simulink model "ej0311_PID"  (R2023b)
settings: Solver=VariableStepAuto  StartTime=0.0  StopTime=30  RelTol=1e-3
libraries: simulink x3
settings Model: Creator=cjuar  LastModifiedBy=cjuar

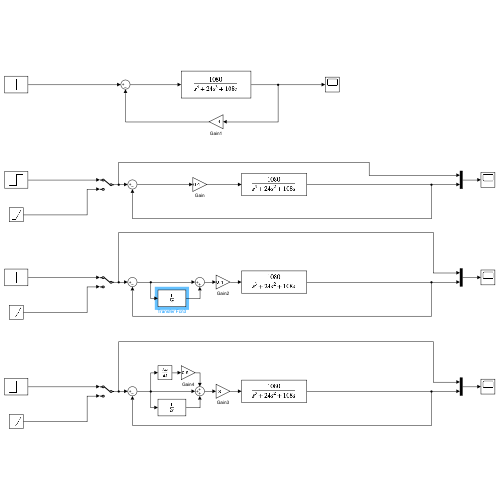
[thumbnail: Simulink's stored preview of the top-level diagram]
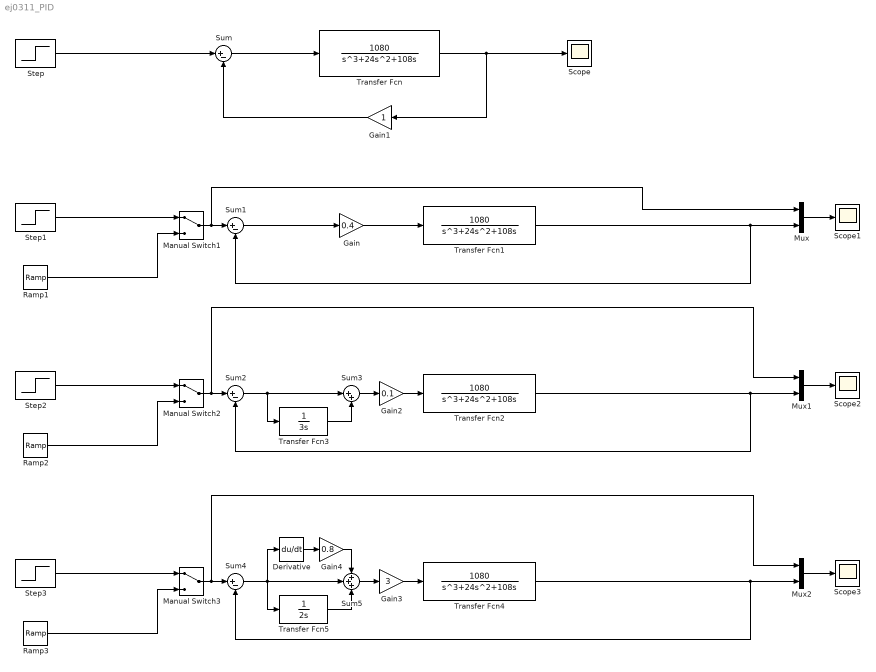
== system ej0311_PID ==
  Derivative : Derivative
  Gain : Gain  Gain=0.4
  Gain1 : Gain
  Gain2 : Gain  Gain=0.1
  Gain3 : Gain  Gain=3
  Gain4 : Gain  Gain=0.8
  Manual Switch1 : ManualSwitch
  Manual Switch2 : ManualSwitch
  Manual Switch3 : ManualSwitch
  Mux : Mux  Inputs=2
  Mux1 : Mux  Inputs=2
  Mux2 : Mux  Inputs=2
  Ramp1 : simulink/Sources/Ramp  slope=1  start=0  InitialOutput=0
  Ramp2 : simulink/Sources/Ramp  slope=1  start=0  InitialOutput=0
  Ramp3 : simulink/Sources/Ramp  slope=1  start=0  InitialOutput=0
  Scope{,1..3} (4 alike) : Scope
  Step{,1..3} (4 alike) : Step  SampleTime=0
  Sum{,1..2,4} (4 alike) : Sum  Inputs=|+-
  Sum3 : Sum  Inputs=|++
  Sum5 : Sum  Inputs=+++
  Transfer Fcn{,1..2,4} (4 alike) : TransferFcn  Numerator=[1080]  Denominator=[1 24 108 0]
  Transfer Fcn3 : TransferFcn  Denominator=[3 0]
  Transfer Fcn5 : TransferFcn  Denominator=[2 0]
  wires:
  Transfer Fcn/1 -> Gain1/1, Scope/1
  Sum/1 -> Transfer Fcn/1
  Transfer Fcn1/1 -> Mux/2, Sum1/2
  Gain/1 -> Transfer Fcn1/1
  Sum1/1 -> Gain/1
  Gain1/1 -> Sum/2
  Step/1 -> Sum/1
  Step1/1 -> Manual Switch1/1
  Ramp1/1 -> Manual Switch1/2
  Manual Switch1/1 -> Mux/1, Sum1/1
  Mux/1 -> Scope1/1
  Mux1/1 -> Scope2/1
  Manual Switch2/1 -> Sum2/1, Mux1/1
  Ramp2/1 -> Manual Switch2/2
  Step2/1 -> Manual Switch2/1
  Gain2/1 -> Transfer Fcn2/1
  Transfer Fcn2/1 -> Sum2/2, Mux1/2
  Sum2/1 -> Transfer Fcn3/1, Sum3/1
  Transfer Fcn3/1 -> Sum3/2
  Sum3/1 -> Gain2/1
  Sum5/1 -> Gain3/1
  Transfer Fcn5/1 -> Sum5/3
  Sum4/1 -> Derivative/1, Sum5/2, Transfer Fcn5/1
  Transfer Fcn4/1 -> Mux2/2, Sum4/2
  Gain3/1 -> Transfer Fcn4/1
  Step3/1 -> Manual Switch3/1
  Ramp3/1 -> Manual Switch3/2
  Manual Switch3/1 -> Mux2/1, Sum4/1
  Mux2/1 -> Scope3/1
  Derivative/1 -> Gain4/1
  Gain4/1 -> Sum5/1
